simulink model "slexResettableSubsystemExample"  (R2019b)
settings: Solver=ode45  StartTime=0.0  StopTime=10.0  FixedStep=.1  RelTol=1e-3  EnableMultiTasking=on
undefined symbols (not defined in the file): DiscIntNeverNeededParam
libraries: simulink x2
Description:
  | Resettable Subsystems
  | 
  | This example shows what happens when a ramp signal is integrated
  | using two resettable subsystems.  After running the simulation, the scope
  | shows three plots.
  | 
  | The middle plot shows the original value of the reset signal.
  | In this example, we are using a discrete sample time pulse signal.
  | The rising and falling edges are what cause the two
  | subsystems to reset.
  | 
  | The top and bottom plots show the original ramp as a reference and its
  | integration. The subsystems corresponding to the top and bottom plots reset on every
  | rising and falling edge of the pulse, respectively.
  | When each subsystem resets, the state of the integrator block is set to its
  | initial condition value, which is 0.
  | You can refer to the middle plot to determine when each subsystem resets.
  | 
  | Notice how the reset happens for blocks within the subsystem,
  | without the need for each block to have its own reset port.
  | This provides a more convenient way of handling reset
  | at a subsystem level.
settings Model: ExtModeTrigMode=oneshot  ExtModeArmWhenConnect=off  ExtModeAutoUpdateStatusClock=off  Creator=The MathWorks, Inc.  LastModifiedBy=bhisma
settings DataIOCC: SaveFormat=StructureWithTime  SaveOutput=off  SaveTime=off
settings OptimizationCC: ExpressionDepthLimit=2147483647  InitFltsAndDblsToZero=on  LifeSpan=inf  BufferReusableBoundary=off
settings DebuggingCC: SaveWithParameterizedLinksMsg=none  SignalResolutionControl=TryResolveAllWithWarning  MultiTaskDSMMsg=warning  MultiTaskCondExecSysMsg=none  IntegerOverflowMsg=none  FcnCallInpInsideContextMsg=warning  BusObjectLabelMismatch=none  AllowSymbolicDim=off  StateNameClashWarn=warning  SFUnexpectedBacktrackingDiag=warning  SFNoUnconditionalDefaultTransitionDiag=warning  SFExecutionAtInitializationDiag=none  IntegerSaturationMsg=none  ArithmeticOperatorsInVariantConditions=warning
settings HardwareCC: ProdBitPerPointer=32  ProdBitPerSizeT=32  ProdBitPerPtrDiffT=32  ProdLargestAtomicFloat=None  ProdIntDivRoundTo=Undefined  ProdEndianess=Unspecified  ProdWordSize=32  ProdHWDeviceType=32-bit Generic  TargetUnknown=on
settings ModelReferenceCC: PropagateSignalLabelsOutOfModel=off
settings SFSimCC: SimUseLocalCustomCode=off  CustomCodeUndefinedFunction=UseInterfaceOnly
settings RTWCC: Description=Generic Real-Time Target  RTWUseLocalCustomCode=off
settings CodeAppCC: StateflowObjectComments=on
settings GRTTargetCC: TargetFcnLib=ansi_tfl_tmw.mat  TargetLangStandard=C89/C90 (ANSI)  GeneratePreprocessorConditionals=Disable all  CombineOutputUpdateFcns=off  GRTInterface=on
settings ConfigComp: CovMetricSettings=d  CovHtmlReporting=on  CovSaveCumulativeToWorkspaceVar=on  CovSaveSingleToWorkspaceVar=on  CovExternalEMLEnable=off  CovSFcnEnable=off

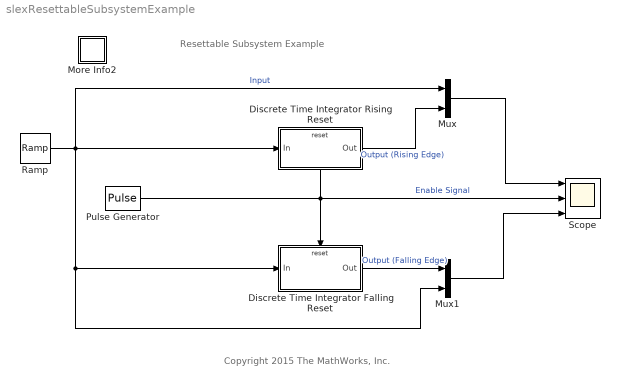
== system slexResettableSubsystemExample ==
  note: Resettable Subsystem Example
  note: Copyright 2015 The MathWorks, Inc.
  Discrete Time Integrator Falling Reset : Subsystem  TreatAsAtomicUnit=on
  Discrete Time Integrator Rising Reset : Subsystem  TreatAsAtomicUnit=on
  More Info2 : Subsystem
      settings: OpenFcn=showdemo(bdroot(gcs))
      mask Display: disp('?')
  Mux : Mux  Inputs=2
  Mux1 : Mux  Inputs=2
  Pulse Generator : DiscretePulseGenerator  Period=40  PulseWidth=20  SampleTime=.1
      settings: AttributesFormatString=Period: %<period>\nDuty cycle: %<pulsewidth>%
  Ramp : simulink/Sources/Ramp  slope=0.5  start=0  InitialOutput=1
  Scope : Scope  NumInputPorts=3
      settings: StartFcn=open_system(gcbh)
  wires:
  Ramp/1 -> Mux/1, Discrete Time Integrator Rising Reset/1(In), Mux1/2, Discrete Time Integrator Falling Reset/1(In)  "Input"
  Discrete Time Integrator Falling Reset/1(Out) -> Mux1/1  "Output (Falling Edge)"
  Discrete Time Integrator Rising Reset/1(Out) -> Mux/2  "Output (Rising Edge)"
  Mux/1 -> Scope/1
  Pulse Generator/1 -> Scope/2, Discrete Time Integrator Falling Reset/Reset, Discrete Time Integrator Rising Reset/Reset  "Enable Signal"
  Mux1/1 -> Scope/3

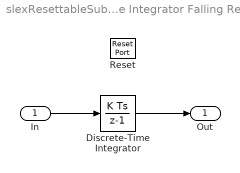
== system slexResettableSubsystemExample/Discrete Time Integrator Falling Reset ==
  In : Inport  SampleTime=.1
  Reset : ResetPort  DisableCoverage=on  ResetTriggerType=falling
  Discrete-Time Integrator : DiscreteIntegrator  SampleTime=.1  ICPrevOutput=DiscIntNeverNeededParam  ICPrevScaledInput=DiscIntNeverNeededParam
  Out : Outport  VectorParamsAs1DForOutWhenUnconnected=off
  wires:
  Discrete-Time Integrator/1 -> Out/1
  In/1 -> Discrete-Time Integrator/1

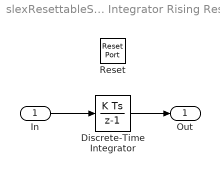
== system slexResettableSubsystemExample/Discrete Time Integrator Rising Reset ==
  In : Inport  SampleTime=0.1
  Reset : ResetPort  DisableCoverage=on
  Discrete-Time Integrator : DiscreteIntegrator  SampleTime=-1  ICPrevOutput=DiscIntNeverNeededParam  ICPrevScaledInput=DiscIntNeverNeededParam
  Out : Outport  OutputWhenDisabled=reset  InitialOutput=0  VectorParamsAs1DForOutWhenUnconnected=off
  wires:
  In/1 -> Discrete-Time Integrator/1
  Discrete-Time Integrator/1 -> Out/1

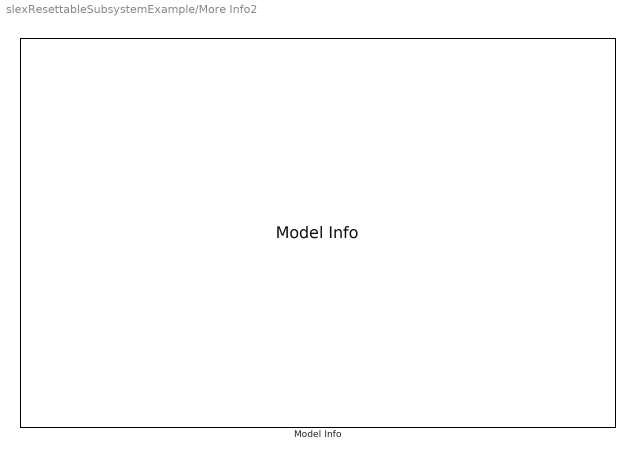
== system slexResettableSubsystemExample/More Info2 ==
  Model Info : simulink/Model-Wide Utilities/Model Info  Frame=on  DisplayStringWithTags=Model Info  HorizontalTextAlignment=Left  LeftAlignmentValue=0.02
